simulink model "Full_car_model_build_Rajesh_Ramani_textbook"  (R2024b)
settings: Solver=VariableStepAuto  StartTime=0.0  StopTime=10  RelTol=1e-3
model workspace: external: MATLAB File C:\Users\USER\Documents\MATLAB\NR\TV_lisb_helper_file.m (data not in the file)
values from neighbouring files (symbols this model uses):
  g = 9.8    [TV_lisb_helper_file.m]
  hCG = 0.6    [TV_lisb_helper_file.m]
  Izz = 3000    [TV_lisb_helper_file.m]
  lf = 1.5    [TV_lisb_helper_file.m]
  lr = 1.5    [TV_lisb_helper_file.m]
  M = 300    [TV_lisb_helper_file.m]
  tr = 1    [TV_lisb_helper_file.m]
libraries: autolibshared x4
(part 4 of 4)

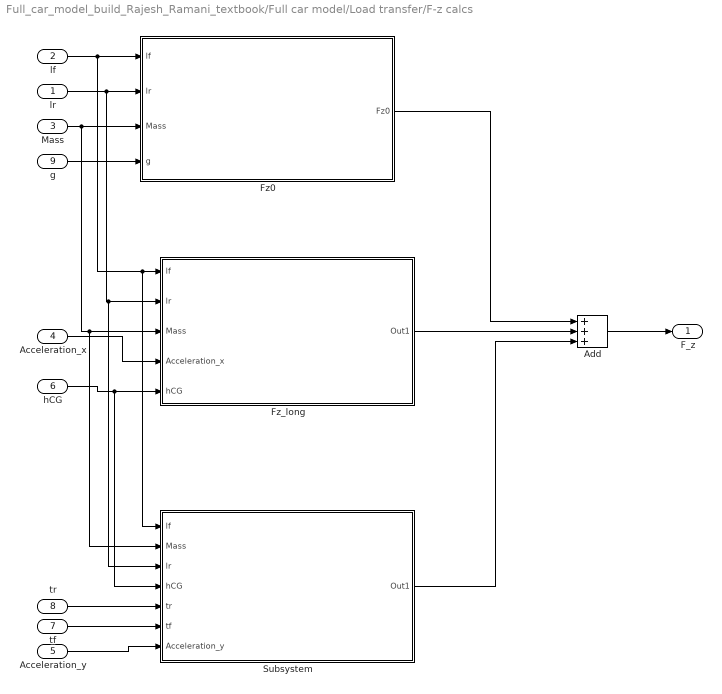
== system Full_car_model_build_Rajesh_Ramani_textbook/Full car model/Load transfer/F-z calcs ==
  lr : Inport
  lf : Inport  Port=2
  Mass : Inport  Port=3
  Acceleration_x : Inport  Port=4
  Acceleration_y : Inport  Port=5
  hCG : Inport  Port=6
  tf : Inport  Port=7
  tr : Inport  Port=8
  g : Inport  Port=9
  Add : Sum  Inputs=+++
  Fz0 : Subsystem
  Fz_long : Subsystem
  Subsystem : Subsystem
  F_z : Outport
  wires:
  Add/1 -> F_z/1
  lf/1 -> Subsystem/1(lf), Fz_long/1(lf), Fz0/1(lf)
  lr/1 -> Subsystem/3(lr), Fz_long/2(lr), Fz0/2(lr)
  g/1 -> Fz0/4(g)
  Mass/1 -> Subsystem/2(Mass), Fz_long/3(Mass), Fz0/3(Mass)
  hCG/1 -> Subsystem/4(hCG), Fz_long/5(hCG)
  Acceleration_x/1 -> Fz_long/4(Acceleration_x)
  Fz0/1(Fz0) -> Add/1
  tr/1 -> Subsystem/5(tr)
  tf/1 -> Subsystem/6(tf)
  Acceleration_y/1 -> Subsystem/7(Acceleration_y)
  Fz_long/1(Out1) -> Add/2
  Subsystem/1(Out1) -> Add/3

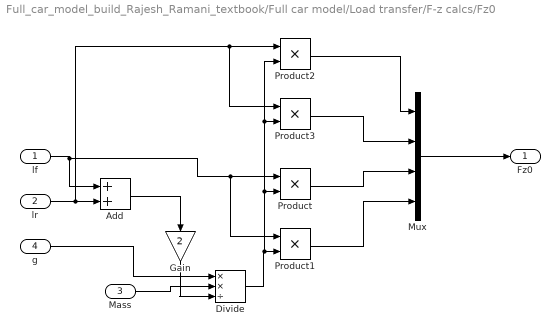
== system Full_car_model_build_Rajesh_Ramani_textbook/Full car model/Load transfer/F-z calcs/Fz0 ==
  lf : Inport
  lr : Inport  Port=2
  Mass : Inport  Port=3
  g : Inport  Port=4
  Add : Sum
  Divide : Product  Inputs=**/
  Gain : Gain  Gain=2
  Mux : Mux
  Product{,1..3} (4 alike) : Product
  Fz0 : Outport
  wires:
  Mass/1 -> Divide/2
  g/1 -> Divide/1
  lr/1 -> Product3/1, Product2/1, Add/2
  lf/1 -> Product1/1, Product/1, Add/1
  Add/1 -> Gain/1
  Gain/1 -> Divide/3
  Mux/1 -> Fz0/1
  Product2/1 -> Mux/1
  Product3/1 -> Mux/2
  Product/1 -> Mux/3
  Product1/1 -> Mux/4
  Divide/1 -> Product2/2, Product3/2, Product/2, Product1/2

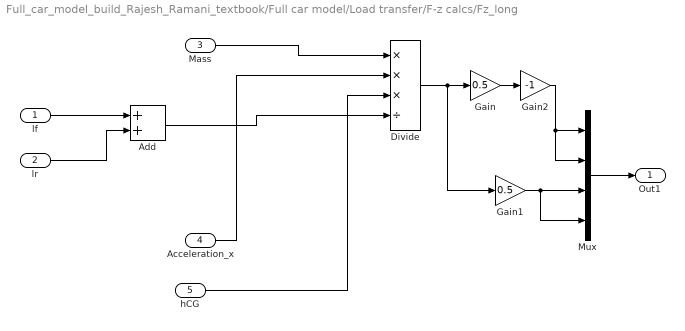
== system Full_car_model_build_Rajesh_Ramani_textbook/Full car model/Load transfer/F-z calcs/Fz_long ==
  lf : Inport
  lr : Inport  Port=2
  Mass : Inport  Port=3
  Acceleration_x : Inport  Port=4
  hCG : Inport  Port=5
  Add : Sum
  Divide : Product  Inputs=***/
  Gain : Gain  Gain=0.5
  Gain1 : Gain  Gain=0.5
  Gain2 : Gain  Gain=-1
  Mux : Mux
  Out1 : Outport
  wires:
  Mass/1 -> Divide/1
  Acceleration_x/1 -> Divide/2
  hCG/1 -> Divide/3
  lr/1 -> Add/2
  lf/1 -> Add/1
  Add/1 -> Divide/4
  Divide/1 -> Gain1/1, Gain/1
  Mux/1 -> Out1/1
  Gain/1 -> Gain2/1
  Gain1/1 -> Mux/4, Mux/3
  Gain2/1 -> Mux/2, Mux/1

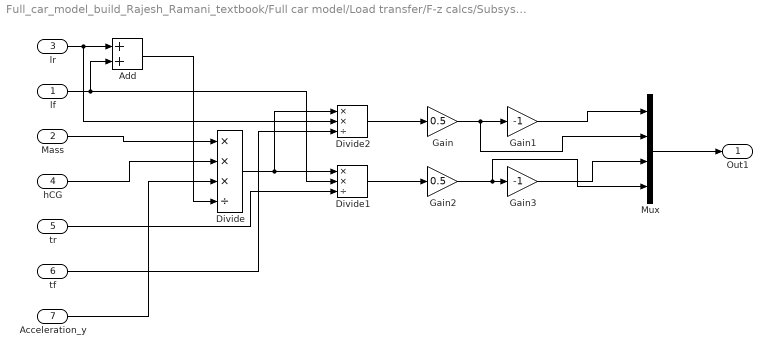
== system Full_car_model_build_Rajesh_Ramani_textbook/Full car model/Load transfer/F-z calcs/Subsystem ==
  lf : Inport
  Mass : Inport  Port=2
  lr : Inport  Port=3
  hCG : Inport  Port=4
  tr : Inport  Port=5
  tf : Inport  Port=6
  Acceleration_y : Inport  Port=7
  Add : Sum
  Divide : Product  Inputs=***/
  Divide1 : Product  Inputs=**/
  Divide2 : Product  Inputs=**/
  Gain : Gain  Gain=0.5
  Gain1 : Gain  Gain=-1
  Gain2 : Gain  Gain=0.5
  Gain3 : Gain  Gain=-1
  Mux : Mux
  Out1 : Outport
  wires:
  Mux/1 -> Out1/1
  Mass/1 -> Divide/1
  hCG/1 -> Divide/2
  Acceleration_y/1 -> Divide/3
  lr/1 -> Divide2/2, Add/1
  lf/1 -> Divide1/2, Add/2
  Add/1 -> Divide/4
  Divide/1 -> Divide2/1, Divide1/1
  tf/1 -> Divide2/3
  Divide2/1 -> Gain/1
  Gain/1 -> Mux/2, Gain1/1
  tr/1 -> Divide1/3
  Gain2/1 -> Mux/4, Gain3/1
  Divide1/1 -> Gain2/1
  Gain1/1 -> Mux/1
  Gain3/1 -> Mux/3
